simulink model "simulate_sensors"  (R2025a)
settings: Solver=FixedStepAuto  StartTime=0.0  StopTime=30  FixedStep=dt_ekf  RelTol=1e-3
model workspace (MATLAB code in the model file):
  | dt_gps = 1/20;
  | dt_imu = 1/200;
  | dt_ekf = 1/100;
undefined symbols (not defined in the file or in its folder): fractalcoef
libraries: mspsensorlib x2, simulink_extras x2, sensorgpslib x1
settings Model: Creator=jonno  LastModifiedBy=jonno

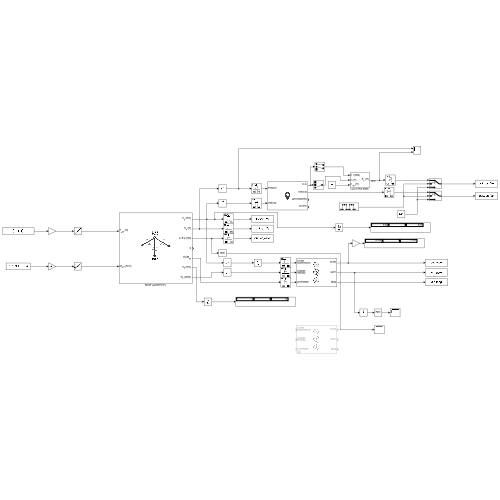
[thumbnail: Simulink's stored preview of the top-level diagram]
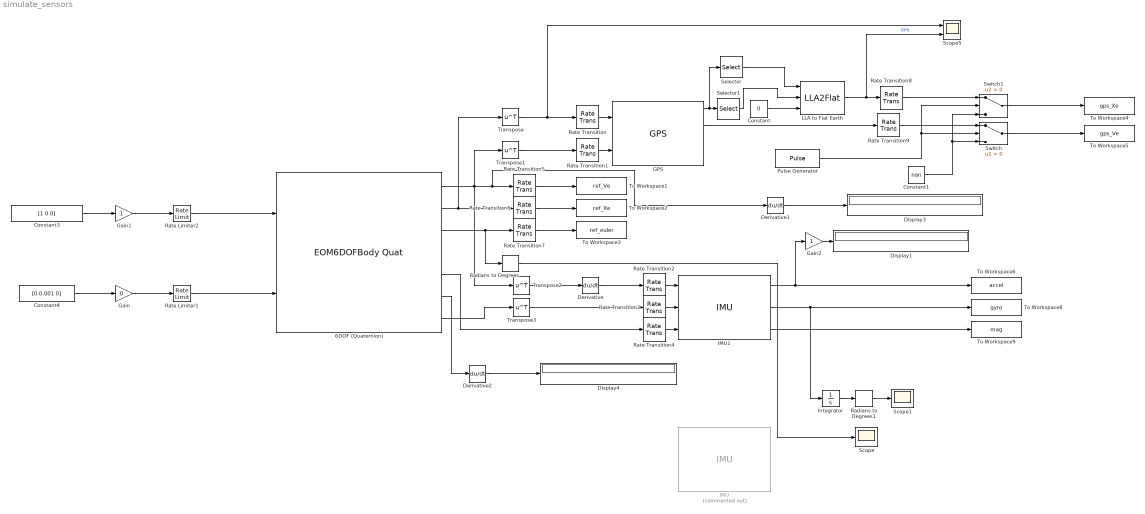
== system simulate_sensors ==
  6DOF (Quaternion) : EOM6DOFBodyQuat  eul_0=[0 +30*pi/180 0]
  Constant : Constant  Value=0
  Constant1 : Constant  Value=nan
  Constant3 : Constant  Value=[1 0 0]
  Constant4 : Constant  Value=[0 0.001 0]
  Derivative : Derivative
  Derivative1 : Derivative
  Derivative2 : Derivative
  Display1 : Display
  Display3 : Display
  Display4 : Display
  GPS : sensorgpslib/GPS  DispRefFrame=NED  PositionInputFormat=Local  ReferenceLocation=[ 0, 0, 0 ]  HorizontalPositionAccuracy=2.5  VerticalPositionAccuracy=3  VelocityAccuracy=0.1  DecayFactor=0.999  SeedDouble=67  SimulateUsing=Interpreted execution
      settings: LibrarySourceBlock=mspsensorlib/GPS
  Gain : Gain  Gain=0
  Gain1 : Gain
  Gain2 : Gain
  IMU : mspsensorlib/IMU  Commented=on  DispRefFrame=NED  TemperaturePort=off  Temperature=25  MagneticFieldPort=off  MagneticFieldNED=[ 27.5550, -2.4169, -16.0849 ]  MagneticFieldENU=[ -2.4169, 27.5550, 16.0849 ]  SeedDouble=67  SimulateUsing=Code generation  AccelParamsMeasurementRange=16*9.81  AccelParamsResolution=((0.732)/1000)*9.81  AccelParamsConstantBias=[0 0.0 0.0]  AccelParamsAxesMisalignment=[0 0 0]  AccelParamsNoiseDensity=[0 0 0]  AccelParamsBiasInstability=[0 0 0]  AccelParamsBiasInstabilityNumerator=fractalcoef().Numerator  AccelParamsBiasInstabilityDenominator=fractalcoef().Denominator  AccelParamsRandomWalk=[0 0 0]  AccelParamsNoiseType=double-sided  AccelParamsTemperatureBias=[0 0 0]  AccelParamsTemperatureScaleFactor=[0 0 0]  GyroParamsMeasurementRange=34.9066  GyroParamsResolution=0.0017453  GyroParamsConstantBias=[0 0 0]  GyroParamsAxesMisalignment=0  GyroParamsAccelerationBias=[0 0 0]  GyroParamsNoiseDensity=[2.9e-4 2.9e-4 2.9e-4]  GyroParamsBiasInstability=[4.8e-5 4.8e-5 4.8e-5]  GyroParamsBiasInstabilityNumerator=fractalcoef().Numerator  GyroParamsBiasInstabilityDenominator=fractalcoef().Denominator  GyroParamsRandomWalk=[0 0 0]  GyroParamsNoiseType=double-sided  GyroParamsTemperatureBias=[0 0 0]  GyroParamsTemperatureScaleFactor=[0 0 0]  MagParamsMeasurementRange=800  MagParamsResolution=0.025  MagParamsConstantBias=0  MagParamsAxesMisalignment=[0 0 0]  MagParamsNoiseDensity=[0 0 0]  MagParamsBiasInstability=[0 0 0]  MagParamsBiasInstabilityNumerator=fractalcoef().Numerator  MagParamsBiasInstabilityDenominator=fractalcoef().Denominator  MagParamsRandomWalk=[0 0 0]  MagParamsNoiseType=double-sided  MagParamsTemperatureBias=[0 0 0]  MagParamsTemperatureScaleFactor=[0 0 0]
  IMU1 : mspsensorlib/IMU  DispRefFrame=NED  TemperaturePort=off  Temperature=25  MagneticFieldPort=off  MagneticFieldNED=[ 27.5550, -2.4169, -16.0849 ]  MagneticFieldENU=[ -2.4169, 27.5550, 16.0849 ]  SeedDouble=67  SimulateUsing=Code generation  AccelParamsMeasurementRange=16*9.81  AccelParamsResolution=((0.732)/1000)*9.81  AccelParamsConstantBias=[0 0.0 0.0]  AccelParamsAxesMisalignment=[0 0 0]  AccelParamsNoiseDensity=[3.9e-3 3.9e-3 3.9e-3].*0  AccelParamsBiasInstability=[5.0e-3 5.0e-3 5.0e-3].*0  AccelParamsBiasInstabilityNumerator=fractalcoef().Numerator  AccelParamsBiasInstabilityDenominator=fractalcoef().Denominator  AccelParamsRandomWalk=[0 0 0]  AccelParamsNoiseType=double-sided  AccelParamsTemperatureBias=[0 0 0]  AccelParamsTemperatureScaleFactor=[0 0 0]  GyroParamsMeasurementRange=34.9066  GyroParamsResolution=0.0017453  GyroParamsConstantBias=[0 0 0]  GyroParamsAxesMisalignment=0  GyroParamsAccelerationBias=[0 0 0]  GyroParamsNoiseDensity=[3.0e-3 3.0e-3 3.0e-3]  GyroParamsBiasInstability=[4.8e-4 4.8e-4 4.8e-4]  GyroParamsBiasInstabilityNumerator=fractalcoef().Numerator  GyroParamsBiasInstabilityDenominator=fractalcoef().Denominator  GyroParamsRandomWalk=[0 0 0]  GyroParamsNoiseType=double-sided  GyroParamsTemperatureBias=[0 0 0]  GyroParamsTemperatureScaleFactor=[0 0 0]  MagParamsMeasurementRange=800  MagParamsResolution=0.025  MagParamsConstantBias=0  MagParamsAxesMisalignment=[0 0 0]  MagParamsNoiseDensity=[0.1 0.1 0.1]  MagParamsBiasInstability=[0 0 0]  MagParamsBiasInstabilityNumerator=fractalcoef().Numerator  MagParamsBiasInstabilityDenominator=fractalcoef().Denominator  MagParamsRandomWalk=[0 0 0]  MagParamsNoiseType=double-sided  MagParamsTemperatureBias=[0 0 0]  MagParamsTemperatureScaleFactor=[0 0 0]
  Integrator : Integrator
  LLA to Flat Earth : LLA2Flat  LL0=[0 0]
  Pulse Generator : DiscretePulseGenerator  Period=dt_gps/dt_ekf  SampleTime=dt_ekf
  Radians to Degrees : simulink_extras/Transformations/Radians to Degrees
  Radians to Degrees1 : simulink_extras/Transformations/Radians to Degrees
  Rate Limiter1 : RateLimiter  SampleTimeMode=inherited
  Rate Limiter2 : RateLimiter  SampleTimeMode=inherited
  Rate Transition{,1..9} (10 alike) : RateTransition  OutPortSampleTime=dt_ekf
  Scope : Scope
      settings: ActiveDisplayYMinimum=-10.419736242536136  ActiveDisplayYMaximum=86.999248894017285
  Scope1 : Scope
      settings: ActiveDisplayYMinimum=-17.490435795984297  ActiveDisplayYMaximum=92.586437441472384
  Scope5 : Scope  NumInputPorts=2
      settings: ActiveDisplayYMinimum=-526.92288558658822  ActiveDisplayYMaximum=4728.54483239818  DataLoggingVariableName=ScopeData5
  Selector : Selector  InputPortWidth=3  IndexOptions=Index vector (dialog)  Indices=[1 2]  OutputSizes=1
  Selector1 : Selector  InputPortWidth=3  IndexOptions=Index vector (dialog)  Indices=[3]  OutputSizes=1
  Switch : Switch  Criteria=u2 > Threshold  SaturateOnIntegerOverflow=off  InputSameDT=off
  Switch1 : Switch  Criteria=u2 > Threshold  SaturateOnIntegerOverflow=off  InputSameDT=off
  To Workspace1 : ToWorkspace  VariableName=ref_Ve  SaveFormat=Timeseries  SampleTime=-1
  To Workspace2 : ToWorkspace  VariableName=ref_Xe  SaveFormat=Timeseries  SampleTime=-1
  To Workspace3 : ToWorkspace  VariableName=ref_euler  SaveFormat=Timeseries  SampleTime=-1
  To Workspace4 : ToWorkspace  VariableName=gps_Xe  SaveFormat=Timeseries  SampleTime=-1
  To Workspace5 : ToWorkspace  VariableName=gps_Ve  SaveFormat=Timeseries  SampleTime=-1
  To Workspace6 : ToWorkspace  VariableName=accel  SaveFormat=Timeseries  SampleTime=-1
  To Workspace8 : ToWorkspace  VariableName=gyro  SaveFormat=Timeseries  SampleTime=-1
  To Workspace9 : ToWorkspace  VariableName=mag  SaveFormat=Timeseries  SampleTime=-1
  Transpose{,1..3} (4 alike) : Math  Operator=transpose
  wires:
  Derivative/1 -> Rate Transition2/1
  6DOF (Quaternion)/7 -> Transpose3/1
  Transpose3/1 -> Rate Transition3/1
  IMU1/2 -> Integrator/1, To Workspace8/1
  GPS/2 -> Rate Transition9/1
  Rate Transition4/1 -> IMU1/3
  Transpose2/1 -> Derivative/1
  LLA to Flat Earth/1 -> Scope5/2, Rate Transition8/1  "GPS"
  Rate Transition2/1 -> IMU1/1
  Constant3/1 -> Gain1/1
  Selector1/1 -> LLA to Flat Earth/2
  Transpose1/1 -> Rate Transition1/1
  Rate Transition1/1 -> GPS/2
  6DOF (Quaternion)/2 -> Rate Transition6/1, Transpose/1
  Rate Transition8/1 -> Switch1/1
  Rate Transition3/1 -> IMU1/2
  Pulse Generator/1 -> Switch/2, Switch1/2
  Rate Transition/1 -> GPS/1
  Selector/1 -> LLA to Flat Earth/1
  Constant/1 -> LLA to Flat Earth/3
  GPS/1 -> Selector/1, Selector1/1
  IMU1/3 -> To Workspace9/1
  Constant1/1 -> Switch1/3, Switch/3
  Rate Transition9/1 -> Switch/1
  Constant4/1 -> Gain/1
  Transpose/1 -> Scope5/1, Rate Transition/1
  6DOF (Quaternion)/5 -> Rate Transition4/1
  Switch1/1 -> To Workspace4/1
  Switch/1 -> To Workspace5/1
  6DOF (Quaternion)/3 -> Radians to Degrees/1, Rate Transition7/1
  Rate Transition5/1 -> To Workspace1/1
  Rate Transition6/1 -> To Workspace2/1
  Rate Transition7/1 -> To Workspace3/1
  IMU1/1 -> Gain2/1, To Workspace6/1
  Gain1/1 -> Rate Limiter2/1
  Rate Limiter1/1 -> 6DOF (Quaternion)/2
  Radians to Degrees/1 -> Scope/1
  Integrator/1 -> Radians to Degrees1/1
  Radians to Degrees1/1 -> Scope1/1
  Gain/1 -> Rate Limiter1/1
  Derivative1/1 -> Display3/1
  Derivative2/1 -> Display4/1
  6DOF (Quaternion)/6 -> Derivative2/1
  Gain2/1 -> Display1/1
  6DOF (Quaternion)/1 -> Transpose2/1, Derivative1/1, Rate Transition5/1, Transpose1/1
  Rate Limiter2/1 -> 6DOF (Quaternion)/1
